simulink model "industrialController"  (R2015b)
settings: Solver=ode3  StartTime=0.0  StopTime=inf  FixedStep=ta  RelTol=1e-3
StopFcn:
  | %serialWrite(0,COMPort,true)
model workspace (MAT data in the model file):
  ta = 0.0333333333333
undefined symbols (not defined in the file or in its folder): DiscIntNeverNeededParam, IsPositionTracked, IsSkeletonTracked, JointDepthIndices, JointImageIndices, JointTrackingState, JointWorldCoordinates, PositionDepthIndices, PositionImageIndices, PositionWorldCoordinates, SegmentationData, SkeletonTrackingID, videoinput
libraries: imaqlib x1, visionsinks x1, simulink x1
settings Model: ExtModeTrigDuration=2  Creator=METZLER  LastModifiedBy=METZLER
settings DataIOCC: SaveFormat=Array
settings OptimizationCC: EfficientMapNaN2IntZero=off  OptimizeModelRefInitCode=on  LifeSpan=1  MaxStackSize=64
settings DebuggingCC: UnderspecifiedInitializationDetection=Classic  MergeDetectMultiDrivingBlocksExec=none
settings HardwareCC: ProdBitPerInt=16  ProdBitPerPointer=16  ProdLargestAtomicFloat=None  ProdWordSize=8  ProdHWDeviceType=Atmel->AVR  TargetBitPerPointer=64  TargetLongLongMode=on  TargetIntDivRoundTo=Zero  TargetEndianess=LittleEndian  TargetWordSize=64  TargetHWDeviceType=MATLAB Host  ProdEqTarget=off
settings CodeAppCC: MaxIdLength=128
settings GRTTargetCC: CombineOutputUpdateFcns=off  GRTInterface=on
settings ConfigComp: CovModelRefEnable=Off

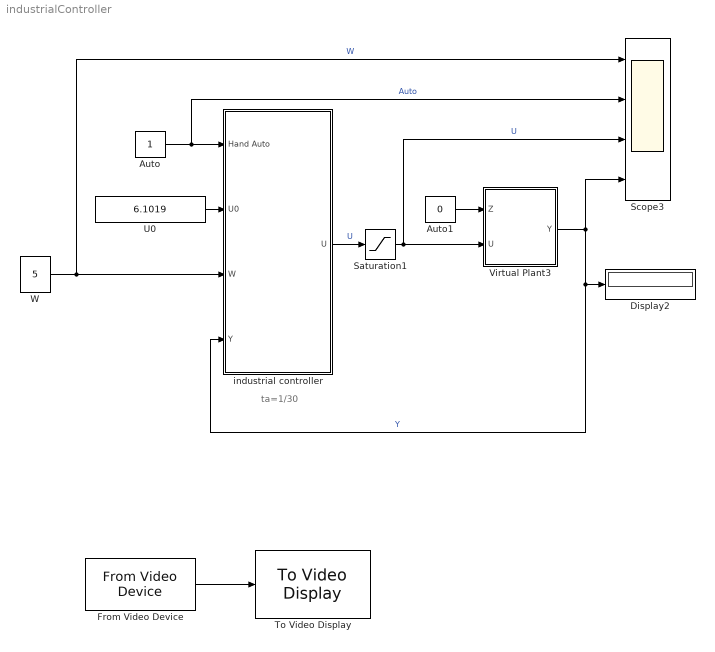
== system industrialController ==
  note: ta=1/30
  Auto : Constant
  Auto1 : Constant  Value=0
  Display2 : Display
  From Video Device : imaqlib/From Video Device  DeviceMenu=winvideo 1 (Integrated Webcam)  Device=winvideo 1 (Microsoft LifeCam HD-3000)  ObjConstructor=videoinput('winvideo', 1)  VideoFormatMenu=MJPG_1280x720  VideoFormat=MJPG_1280x720  VideoSource=input1  ROIPosition=[0 0 720 1280]  EnableHWTrigger=off  TriggerConfiguration=winvideo 1 (Microsoft LifeCam HD-3000)  SampleTime=1/30  OutputPortsMode=One multidimensional signal  DataType=single  CanDoHWTrigger=no  ReturnedColorSpace=rgb  BlockHandle=2292.0004  ROIWidth=1280  ROIHeight=720  ROIColumn=0  ROIRow=0  EngXMLPath=C:\Program Files\MATLAB\R2015b\toolbox\imaq\imaq\private  DevXMLPath=C:\MATLAB\SupportPackages\R2015b\osgenericvideointerface\toolbox\imaq\supportpackages\genericvideo\adaptor\win64  EngLibPath=C:\Program Files\MATLAB\R2015b\toolbox\imaq\imaqblks\imaqmex\win64  ColorSpace=rgb  BayerSensorAlignment=grbg  AllMetadata=IsPositionTracked;IsSkeletonTracked;JointDepthIndices;JointImageIndices;JointTrackingState;JointWorldCoordinates;PositionDepthIndices;PositionImageIndices;PositionWorldCoordinates;SegmentationData;SkeletonTrackingID
  Saturation1 : Saturate  UpperLimit=7.5  LowerLimit=4.5
      settings: AttributesFormatString=|
      | Lower Limit=%<LowerLimit>
      | Upper Limit=%<UpperLimit>
  Scope3 : Scope  NumInputPorts=4
  To Video Display : visionsinks/To Video Display  windowSizeMode=Normal  openAtMdlStart=on  fullScreen=off  videoWindowX=536805376  videoWindowY=536805376  saveWindowSize=off  videoWindowWidth=1280  videoWindowHeight=720  inputColorFormat=RGB  inputType=Obsolete  imagePorts=One multidimensional signal  OutputDevice=On-screen video monitor  dataOrg=Column-major  isWindowOpen=off
  U0 : Constant  Value=6.1019
  Virtual Plant3 : Subsystem
  W : Constant  Value=5
  industrial controller : Subsystem  mask{kpr=0.7702, kir=0.1621, kdr=0.8783, RemoveInitialError=1, T=0.1}
      mask prompts: kpr "cpc (Constant Proportional Controler)"; kir "cic (Constant Integral Controler)"; kdr "cdc (Constant Derivative Controller)"; RemoveInitialError "Initial Error (0 for keeping, 1 for removing)"; T "T (Time Constant of Real D-Block)"
      mask help: Industrial Controller for Mooc MSUS
      mask Display:
      | port_label('input',1,'Hand->Automatic');
      | port_label('input',2,'U0');
      | port_label('input',3,'W');
      | port_label('input',4,'Y');
      | port_label('output',1,'U');
  wires:
  industrial controller/1(U) -> Saturation1/1  "U"
  U0/1 -> industrial controller/2(U0)
  W/1 -> Scope3/1, industrial controller/3(W)  "W"
  Auto/1 -> industrial controller/1(Hand Auto), Scope3/2  "Auto"
  Saturation1/1 -> Scope3/3, Virtual Plant3/2(U)  "U"
  Virtual Plant3/1(Y) -> Scope3/4, industrial controller/4(Y), Display2/1  "Y"
  Auto1/1 -> Virtual Plant3/1(Z)
  From Video Device/1 -> To Video Display/1

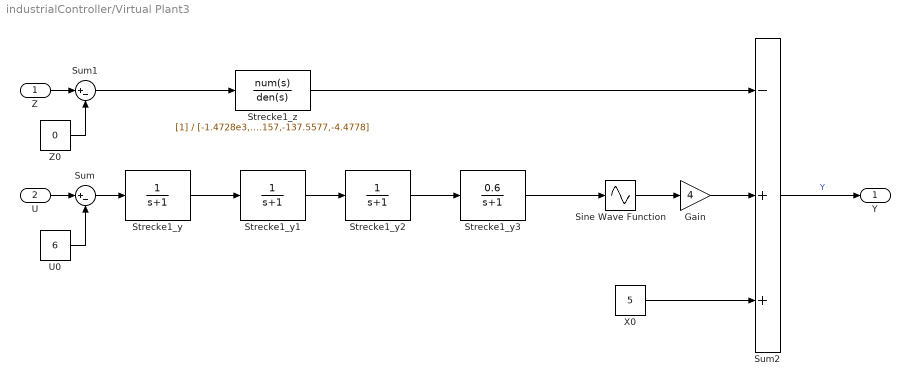
== system industrialController/Virtual Plant3 ==
  Z : Inport
  U : Inport  Port=2
  Gain : Gain  Gain=4
  Sine Wave Function : Sin  TimeSource=Use external signal  SampleTime=0
  Strecke1_y : TransferFcn  Denominator=[1,1]
  Strecke1_y1 : TransferFcn  Denominator=[1,1]
  Strecke1_y2 : TransferFcn  Denominator=[1,1]
  Strecke1_y3 : TransferFcn  Numerator=[0.6]  Denominator=[1,1]
  Strecke1_z : TransferFcn  Denominator=[-1.4728e3,-534.157,-137.5577,-4.4778]
  Sum : Sum  Inputs=|+-
  Sum1 : Sum  Inputs=|+-
  Sum2 : Sum  Inputs=-++
  U0 : Constant  Value=6
  X0 : Constant  Value=5
  Z0 : Constant  Value=0
  Y : Outport
  wires:
  Sum2/1 -> Y/1  "Y"
  U/1 -> Sum/1
  Z/1 -> Sum1/1
  X0/1 -> Sum2/3
  Strecke1_z/1 -> Sum2/1
  Z0/1 -> Sum1/2
  Sum1/1 -> Strecke1_z/1
  U0/1 -> Sum/2
  Sum/1 -> Strecke1_y/1
  Strecke1_y/1 -> Strecke1_y1/1
  Strecke1_y1/1 -> Strecke1_y2/1
  Strecke1_y2/1 -> Strecke1_y3/1
  Strecke1_y3/1 -> Sine Wave Function/1
  Sine Wave Function/1 -> Gain/1
  Gain/1 -> Sum2/2

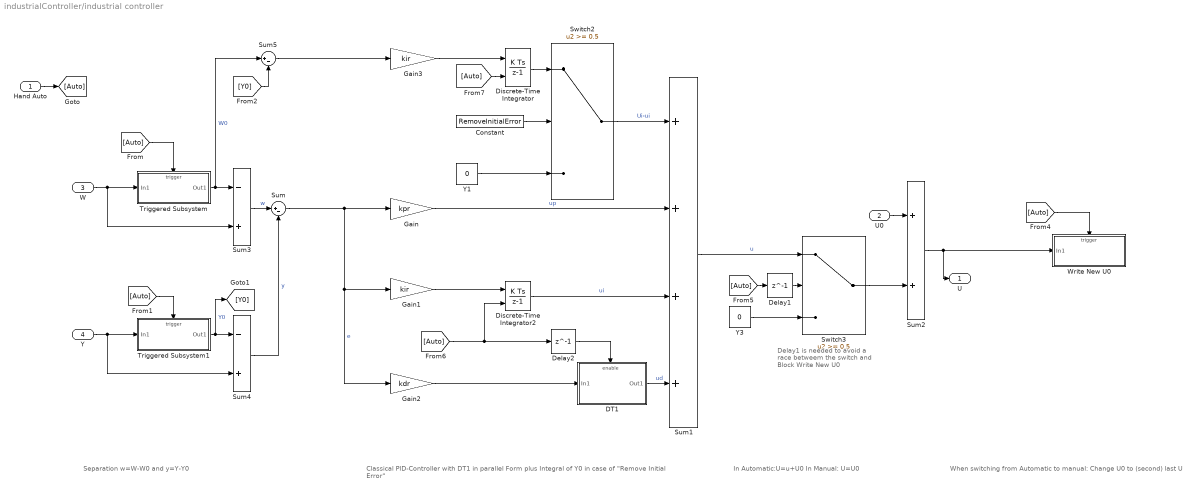
== system industrialController/industrial controller ==
  note: Delay1 is needed to avoid a race betweem the switch and Block Write New U0
  note: Separation w=W-W0
      | and y=Y-Y0
  note: Classical PID-Controller with DT1 in parallel Form
      | plus Integral of Y0 in case of "Remove Initial Error"
  note: In Automatic:U=u+U0
      | In Manual: U=U0
  note: When switching from Automatic to manual:
      | Change U0 to (second) last U
  Hand Auto : Inport
  U0 : Inport  Port=2
  W : Inport  Port=3
  Y : Inport  Port=4
  Constant : Constant  Value=RemoveInitialError
  DT1 : Subsystem
  Delay1 : Delay  DelayLength=1
  Delay2 : Delay  DelayLength=1
  Discrete-Time Integrator : DiscreteIntegrator  ExternalReset=rising  SampleTime=ta  ICPrevOutput=DiscIntNeverNeededParam  ICPrevScaledInput=DiscIntNeverNeededParam
  Discrete-Time Integrator2 : DiscreteIntegrator  ExternalReset=rising  SampleTime=ta  ICPrevOutput=DiscIntNeverNeededParam  ICPrevScaledInput=DiscIntNeverNeededParam
  Gain : Gain  Gain=kpr
  Gain1 : Gain  Gain=kir
  Gain2 : Gain  Gain=kdr
  Gain3 : Gain  Gain=kir
  Sum : Sum  Inputs=|+-
  Sum1 : Sum  Inputs=++++
  Sum2 : Sum
  Sum3 : Sum  Inputs=-+
  Sum4 : Sum  Inputs=-+
  Sum5 : Sum  Inputs=|+-
  Switch2 : Switch  Threshold=0.5
  Switch3 : Switch  Threshold=0.5
  Triggered Subsystem : Subsystem  TreatAsAtomicUnit=on
  Triggered Subsystem1 : Subsystem  TreatAsAtomicUnit=on
  Write New U0 : Subsystem  TreatAsAtomicUnit=on
  Y1 : Constant  Value=0
  Y3 : Constant  Value=0
  U : Outport
  wires:
  Discrete-Time Integrator2/1 -> Sum1/3  "ui"
  Discrete-Time Integrator/1 -> Switch2/1
  Switch2/1 -> Sum1/1  "Ui-ui"
  Constant/1 -> Switch2/2
  Y1/1 -> Switch2/3
  [Y0] -> Sum5/2
  Sum5/1 -> Gain3/1
  Gain3/1 -> Discrete-Time Integrator/1
  Gain/1 -> Sum1/2  "up"
  U0/1 -> Sum2/1
  Hand Auto/1 -> [Auto]
  Sum1/1 -> Switch3/1  "u"
  Sum/1 -> Gain2/1, Gain1/1, Gain/1  "e"
  Gain1/1 -> Discrete-Time Integrator2/1
  [Auto] -> Triggered Subsystem1/Trigger
  [Auto] -> Triggered Subsystem/Trigger
  Triggered Subsystem1/1(Out1) -> [Y0], Sum4/1  "Y0"
  Sum4/1 -> Sum/2  "y"
  Y/1 -> Triggered Subsystem1/1(In1), Sum4/2
  Triggered Subsystem/1(Out1) -> Sum5/1, Sum3/1  "W0"
  Sum3/1 -> Sum/1  "w"
  W/1 -> Triggered Subsystem/1(In1), Sum3/2
  [Auto] -> Write New U0/Trigger
  Y3/1 -> Switch3/3
  [Auto] -> Delay1/1
  Switch3/1 -> Sum2/2
  Sum2/1 -> Write New U0/1(In1), U/1
  [Auto] -> Discrete-Time Integrator2/2, Delay2/1
  [Auto] -> Discrete-Time Integrator/2
  Gain2/1 -> DT1/1(In1)
  DT1/1(Out1) -> Sum1/4  "ud"
  Delay1/1 -> Switch3/2
  Delay2/1 -> DT1/Enable

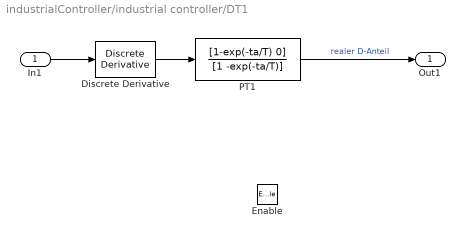
== system industrialController/industrial controller/DT1 ==
  In1 : Inport
  Enable : EnablePort
  Discrete Derivative : simulink/Discrete/Discrete Derivative  gainval=1.0  ICPrevScaledInput=0.0  InputProcessing=Inherited  OutMin=[]  OutMax=[]  OutDataType=fixdt(1, 16)  OutScaling=2^-10  DoSatur=off
  PT1 : DiscreteTransferFcn  Numerator=[1-exp(-ta/T) 0]  Denominator=[1 -exp(-ta/T)]  SampleTime=ta
  Out1 : Outport
  wires:
  In1/1 -> Discrete Derivative/1
  PT1/1 -> Out1/1  "realer D-Anteil"
  Discrete Derivative/1 -> PT1/1

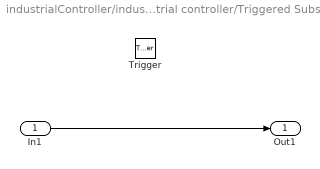
== system industrialController/industrial controller/Triggered Subsystem ==
  In1 : Inport
  Trigger : TriggerPort
  Out1 : Outport
  wires:
  In1/1 -> Out1/1

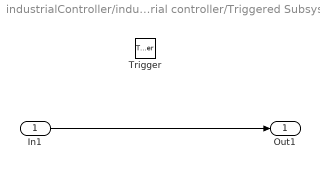
== system industrialController/industrial controller/Triggered Subsystem1 ==
  In1 : Inport
  Trigger : TriggerPort
  Out1 : Outport
  wires:
  In1/1 -> Out1/1

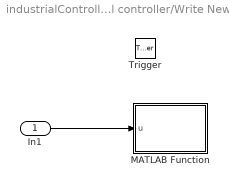
== system industrialController/industrial controller/Write New U0 ==
  In1 : Inport
  Trigger : TriggerPort  TriggerType=falling
  MATLAB Function : MATLAB Function  TreatAsAtomicUnit=on
  wires:
  In1/1 -> MATLAB Function/1(u)

== matlab function industrialController/industrial controller/Write New U0/MATLAB Function ==
  data: u input
function  fcn(u)
%#codegen
coder.extrinsic('set_param')
coder.extrinsic('num2str')
coder.extrinsic('bdroot')
coder.extrinsic('get_param')
coder.extrinsic('gcbh')
coder.extrinsic('gcb')
coder.extrinsic('findstr')
coder.extrinsic('length')
%My_ModelWorkSpace = get_param('C1','ModelWorkSpace')
%My_ModelWorkSpace.assignin('U0', u)
%An awefull lot of code just to move two hirachy steps up...
string='This is just a string that is considered to have enough characters for whatever we want to do with the variable test later down the road let us add somme additional characters like abcdefg and hope that this is enough right now This is just a string that is considered to have enough characters for whatever we want to do with the variable test later down the road let us add somme additional characters like abcdefg and hope that this is enough right now This is just a string that is considered to have enough characters for whatever we want to do with the variable test later down the road let us add somme additional characters like abcdefg and hope that this is enough right now This is just a string that is considered to have enough characters for whatever we want to do with the variable test later down the road let us add somme additional characters like abcdefg and hope that this is enough right now This is just a string that is considered to have enough characters for whatever we want to do with the variable test later down the road let us add somme additional characters like abcdefg and hope that this is enough right now This is just a string that is considered to have enough characters for whatever we want to do with the variable test later down the road let us add somme additional characters like abcdefg and hope that this is enough right now This is just a string that is considered to have enough characters for whatever we want to do with the variable test later down the road let us add somme additional characters like abcdefg and hope that this is enough right now This is just a string that is considered to have enough characters for whatever we want to do with the variable test later down the road let us add somme additional characters like abcdefg and hope that this is enough right now'
Length=uint8(1)
Length=uint8(length(gcb))
string(1:Length)=gcb
index=uint8(1)
index=uint8(strfind(gcb,'industrial controller'))
set_param([string(1:index-1),'U0'],'Value',num2str(u))
end
